simulink model "bh_lag_LQI_eom_quad_include_spin_props"  (R2021b)
settings: Solver=ode23t  StartTime=0.0  StopTime=200  FixedStep=0.001  RelTol=1e-5  EnableMultiTasking=on
values from neighbouring files (symbols this model uses):
  K = [1.17115605021e-19 -1.34457008772e-16 -7.12795123873e-18 0.0431836511993 -1.6541551896e-12 -1.73191982917e-16 0.126584124772 -3.94383892487e-18 1.65419671556e-12 0.126584124772 -1.82762947107e-16 -8.51651764895e-17 ... (60 elements, 4x15)]    [OLD_bh_CONT_DES_RESULTS_LQI_quadcopter.mat]    (also in bh_CONT_DES_RESULTS_LQI_quadcopter.mat = [2.6635655919e-18 -4.41749299763e-16 -1.11640474601e-16 0.04)
undefined symbols (not defined in the file or in its folder): P_elec, P_mot, P_one_prop, P_veh, sigbuilder_block
libraries: bh_6dof_LIBRARY x21, simulink_extras x12, slpidlib x4, simulink x1
(part 2 of 2)

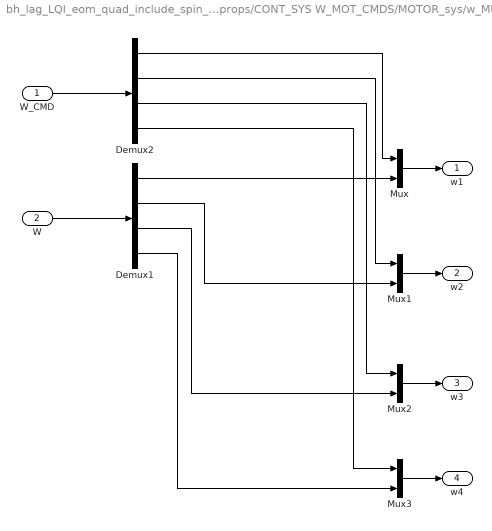
== system bh_lag_LQI_eom_quad_include_spin_props/CONT_SYS W_MOT_CMDS/MOTOR_sys/w_MUX ==
  W_CMD : Inport
  W : Inport  Port=2
  Demux1 : Demux
  Demux2 : Demux
  Mux{,1..3} (4 alike) : Mux  Inputs=2
  w1 : Outport  VectorParamsAs1DForOutWhenUnconnected=off
  w2 : Outport  Port=2  VectorParamsAs1DForOutWhenUnconnected=off
  w3 : Outport  Port=3  VectorParamsAs1DForOutWhenUnconnected=off
  w4 : Outport  Port=4  VectorParamsAs1DForOutWhenUnconnected=off
  wires:
  W_CMD/1 -> Demux2/1
  W/1 -> Demux1/1
  Mux/1 -> w1/1
  Mux1/1 -> w2/1
  Mux3/1 -> w4/1
  Mux2/1 -> w3/1
  Demux2/1 -> Mux/1
  Demux2/2 -> Mux1/1
  Demux2/3 -> Mux2/1
  Demux2/4 -> Mux3/1
  Demux1/1 -> Mux/2
  Demux1/2 -> Mux1/2
  Demux1/3 -> Mux2/2
  Demux1/4 -> Mux3/2

== system bh_lag_LQI_eom_quad_include_spin_props/CONT_SYS W_MOT_CMDS/MOTOR_sys/MOTOR_1/prefilter ==
  note: Y = U *     wn^2/( s^2 + 2*p*wn*s + wn^2)
      | Y*( s^2 + 2*p*wn*s + wn^2) = U * wn^2
      |
      | y'' + y'*2*p*wn + y*wn^2 = U*wn^2
  U : Inport
  Gain : Gain  Gain=2*p*wn
  Gain1 : Gain  Gain=wn^2
  Gain2 : Gain  Gain=wn^2
  Integrator : Integrator
  Integrator1 : Integrator
  Sum : Sum  Inputs=|+--
  U_filt : Outport  VectorParamsAs1DForOutWhenUnconnected=off
  U_DOT : Outport  Port=2  VectorParamsAs1DForOutWhenUnconnected=off
  wires:
  Integrator/1 -> Integrator1/1, [Y_DOT], Gain/1  "y_dot"
  Sum/1 -> Integrator/1  "y_dot_dot"
  Integrator1/1 -> Gain1/1, U_filt/1  "y"
  U/1 -> Gain2/1
  Gain2/1 -> Sum/1
  Gain/1 -> Sum/3
  Gain1/1 -> Sum/2
  [Y_DOT] -> U_DOT/1

== system bh_lag_LQI_eom_quad_include_spin_props/CONT_SYS W_MOT_CMDS/MOTOR_sys/MOTOR_2/prefilter ==
  note: Y = U *     wn^2/( s^2 + 2*p*wn*s + wn^2)
      | Y*( s^2 + 2*p*wn*s + wn^2) = U * wn^2
      |
      | y'' + y'*2*p*wn + y*wn^2 = U*wn^2
  U : Inport
  Gain : Gain  Gain=2*p*wn
  Gain1 : Gain  Gain=wn^2
  Gain2 : Gain  Gain=wn^2
  Integrator : Integrator
  Integrator1 : Integrator
  Sum : Sum  Inputs=|+--
  U_filt : Outport  VectorParamsAs1DForOutWhenUnconnected=off
  U_DOT : Outport  Port=2  VectorParamsAs1DForOutWhenUnconnected=off
  wires:
  Integrator/1 -> Integrator1/1, [Y_DOT], Gain/1  "y_dot"
  Sum/1 -> Integrator/1  "y_dot_dot"
  Integrator1/1 -> Gain1/1, U_filt/1  "y"
  U/1 -> Gain2/1
  Gain2/1 -> Sum/1
  Gain/1 -> Sum/3
  Gain1/1 -> Sum/2
  [Y_DOT] -> U_DOT/1

== system bh_lag_LQI_eom_quad_include_spin_props/CONT_SYS W_MOT_CMDS/MOTOR_sys/MOTOR_3/prefilter ==
  note: Y = U *     wn^2/( s^2 + 2*p*wn*s + wn^2)
      | Y*( s^2 + 2*p*wn*s + wn^2) = U * wn^2
      |
      | y'' + y'*2*p*wn + y*wn^2 = U*wn^2
  U : Inport
  Gain : Gain  Gain=2*p*wn
  Gain1 : Gain  Gain=wn^2
  Gain2 : Gain  Gain=wn^2
  Integrator : Integrator
  Integrator1 : Integrator
  Sum : Sum  Inputs=|+--
  U_filt : Outport  VectorParamsAs1DForOutWhenUnconnected=off
  U_DOT : Outport  Port=2  VectorParamsAs1DForOutWhenUnconnected=off
  wires:
  Integrator/1 -> Integrator1/1, [Y_DOT], Gain/1  "y_dot"
  Sum/1 -> Integrator/1  "y_dot_dot"
  Integrator1/1 -> Gain1/1, U_filt/1  "y"
  U/1 -> Gain2/1
  Gain2/1 -> Sum/1
  Gain/1 -> Sum/3
  Gain1/1 -> Sum/2
  [Y_DOT] -> U_DOT/1

== system bh_lag_LQI_eom_quad_include_spin_props/CONT_SYS W_MOT_CMDS/MOTOR_sys/MOTOR_4/prefilter ==
  note: Y = U *     wn^2/( s^2 + 2*p*wn*s + wn^2)
      | Y*( s^2 + 2*p*wn*s + wn^2) = U * wn^2
      |
      | y'' + y'*2*p*wn + y*wn^2 = U*wn^2
  U : Inport
  Gain : Gain  Gain=2*p*wn
  Gain1 : Gain  Gain=wn^2
  Gain2 : Gain  Gain=wn^2
  Integrator : Integrator
  Integrator1 : Integrator
  Sum : Sum  Inputs=|+--
  U_filt : Outport  VectorParamsAs1DForOutWhenUnconnected=off
  U_DOT : Outport  Port=2  VectorParamsAs1DForOutWhenUnconnected=off
  wires:
  Integrator/1 -> Integrator1/1, [Y_DOT], Gain/1  "y_dot"
  Sum/1 -> Integrator/1  "y_dot_dot"
  Integrator1/1 -> Gain1/1, U_filt/1  "y"
  U/1 -> Gain2/1
  Gain2/1 -> Sum/1
  Gain/1 -> Sum/3
  Gain1/1 -> Sum/2
  [Y_DOT] -> U_DOT/1

== matlab function bh_lag_LQI_eom_quad_include_spin_props/CONT_SYS W_MOT_CMDS/FM_to_w2 ==
  data: L input; w2_cmd output; Thrust_const input; Twist_const input; Thrust input; TQ_roll_X input; TQ_pit_Y input; TQ_yaw_Z input
function w2_cmd = FMtow2(L, Thrust_const, Twist_const, Thrust, TQ_roll_X, TQ_pit_Y, TQ_yaw_Z)
%#codegen

    % simplify the variable names
    b = Thrust_const;
    k = Twist_const;

    % construct the co-efficient matrix:
    %  F_and_M = C * w^2
    %
    C = [     b,    b,    b,    b;
              0,    b*L,  0,   -b*L;
             -b*L,  0,    b*L,  0;
             -k,    k,   -k,    k; ];

    % used Symbolic toolbox to compute inv(C)
    C_inv = [
             1/(4*b),          0, -1/(2*L*b), -1/(4*k);
             1/(4*b),  1/(2*L*b),          0,  1/(4*k);
             1/(4*b),          0,  1/(2*L*b), -1/(4*k);
             1/(4*b), -1/(2*L*b),          0,  1/(4*k);
            ];
    % solve for the w^2 vec
    F_and_M_col = [Thrust, TQ_roll_X, TQ_pit_Y, TQ_yaw_Z].' ;
    w2_cmd      = C_inv * F_and_M_col; 
    
    % check that ALL w^2 >=0
    tf_col      = (w2_cmd >= 0);
%     if( ~all(tf_col) )
%         w2_cmd = lsqnonneg(C, F_and_M_col);
%     end
%     
%     tf_again_col = (w2_cmd >= 0);
%     assert(all(tf_again_col), 'ERROR: ohh dear some w2 are NEGATIVE !')
   
%     for kk=1:4
%       fprintf('\n ... [%.16f]', w2_cmd(kk) );
%     end
%     fprintf('\n -----------------------------------------------');
    assert(all(tf_col), 'ERROR: ohh dear some w2 are NEGATIVE !')
    
% 
%      if( ~all(tf_col) )
%        fprintf('\n ..... WHAT HAPPENED !');
%      end
%     assert(all(tf_col), 'ERROR: ohh dear some w2 are NEGATIVE !')
   %assert(false, 'ERROR: some w2 are NEGATIVE !')
end

== matlab function bh_lag_LQI_eom_quad_include_spin_props/a_circle1/MATLAB Function ==
  data: t_clock input; XYZ output; t_to_start input; RADIUS input; ztgt input; w input
function XYZ = fcn(t_clock, t_to_start, RADIUS, ztgt, w)

t    = t_clock - t_to_start;

theta = w*t;

x = RADIUS * cos(theta);
y = RADIUS * sin(theta);
z = ztgt;


XYZ = [x;y;z];

== matlab function bh_lag_LQI_eom_quad_include_spin_props/CONT_SYS W_MOT_CMDS/w2toFM1 ==
  data: L input; Tbz_col output; Thrust_const input; Twist_const input; w2_col input; Mbz_col output; wM_col output
function [Tbz_col, Mbz_col, wM_col] = w2toFM(L, Thrust_const, Twist_const, w2_col)
%#codegen

    % simplify the variable names
    b = Thrust_const;
    k = Twist_const;

    % construct the co-efficient matrix:
    %  F_and_M = C * w^2
    
%     C = [     b,    b,    b,    b;
%               0,    b*L,  0,   -b*L;
%              -b*L,  0,    b*L,  0;
%              -k,    k,   -k,    k; ];

    Tbz_col = [ b; b; b; b ]  .*  w2_col;     
    Mbz_col = [-k; k;-k; k ]  .*  w2_col;          
    wM_col  = [ 1;-1; 1;-1 ]  .*  sqrt(w2_col); 
end

== matlab function bh_lag_LQI_eom_quad_include_spin_props/CONT_SYS W_MOT_CMDS/w2toFM2 ==
  data: L input; Thrust output; Thrust_const input; Twist_const input; w2_col input; TQ_roll_X output; TQ_pit_Y output; TQ_yaw_Z output
function [Thrust, TQ_roll_X, TQ_pit_Y, TQ_yaw_Z] = w2toFM(L, Thrust_const, Twist_const, w2_col)
%#codegen

    % simplify the variable names
    b = Thrust_const;
    k = Twist_const;

    % construct the co-efficient matrix:
    %  F_and_M = C * w^2
    
    C = [     b,    b,    b,    b;
              0,    b*L,  0,   -b*L;
             -b*L,  0,    b*L,  0;
             -k,    k,   -k,    k; ];

    % solve for the FM_col
    %   FM_col = [Thrust, TQ_roll_X, TQ_pit_Y, TQ_yaw_Z].' ;
    
    FM_col  =  C * w2_col;
    
    Thrust    =  FM_col(1);
    TQ_roll_X =  FM_col(2);
    TQ_pit_Y  =  FM_col(3);
    TQ_yaw_Z  =  FM_col(4);
    
end
